simulink model "top_level_European_4segs_SR"  (R2025b)
settings: Solver=FixedStepAuto  StartTime=0.0  StopTime=tstop-Ts  RelTol=1e-3
undefined symbols (not defined in the file): DiscIntNeverNeededParam, dt, freq, idxC1, idxC2, idxC3, idxC4, n1, n2, n3, n4, Ts
libraries: eeRmsMeasurement x3
settings Model: SimulationMode=accelerator  Creator=gdudgeon  LastModifiedBy=gdudgeon
settings ModelReferenceCC: UpdateModelReferenceTargets=AssumeUpToDate  ParallelModelReferenceMATLABWorkerInit=Copy Base Workspace

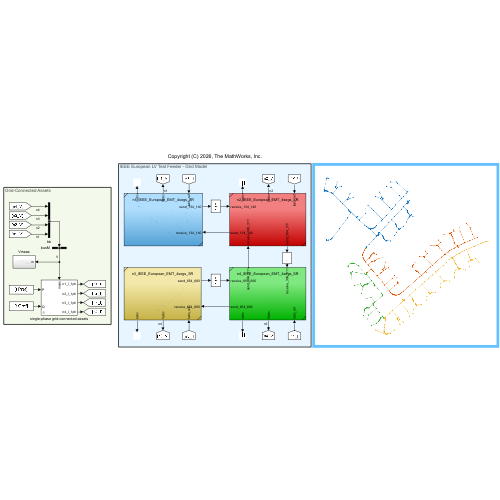
[thumbnail: Simulink's stored preview of the top-level diagram]
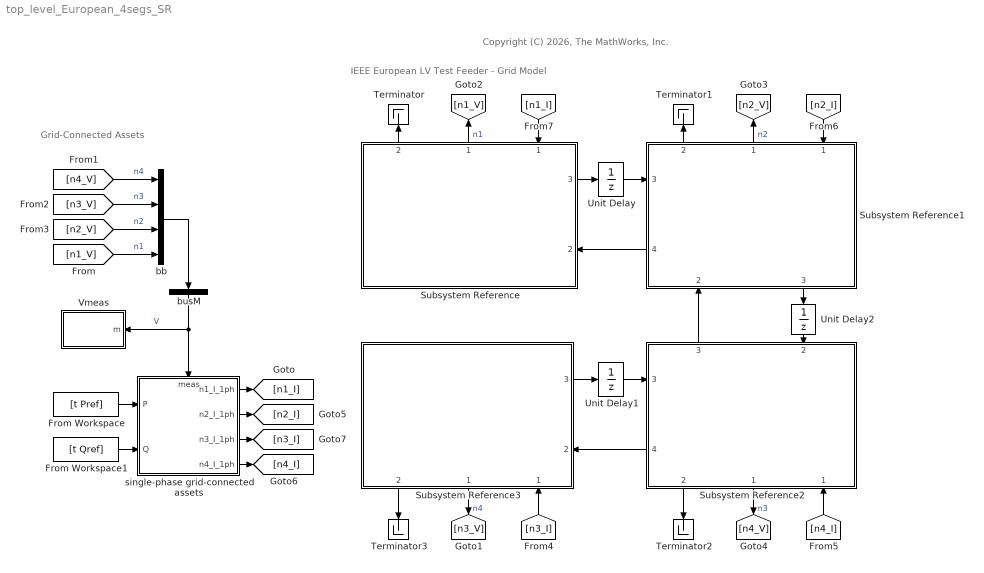
== system top_level_European_4segs_SR ==
  note: IEEE European LV Test Feeder - Grid Model
  note: Grid-Connected Assets
  note: Copyright (C) 2026, The MathWorks, Inc.
  From Workspace : FromWorkspace  VariableName=[t Pref]  SampleTime=Ts
  From Workspace1 : FromWorkspace  VariableName=[t Qref]  SampleTime=Ts
  Subsystem Reference : Subsystem  ReferencedSubsystem=n1_IEEE_European_EMT_4segs_SR
      settings: PortSchema="{\"entries\":[{\"content\":{\"sides\":[{\"content\":{},\"type\":\"ConnectorPlacement.EquallySpacedRectSide\",\"uuid\":\"0602a24e-b238-4b3f-aac8-5c5202892abf\"},{\"content\":{\"connectorIds\":[\"Out3\",\"In2\"],\"side\":\"RIGHT\"},\"type\":\"ConnectorPlacement.EquallySpacedRectSide\",\"uuid\":\"14efc789-be57-4299-a3a5-1e5073bae767\"},{\"content\":{\"connectorIds\":[\"Out2\",\"Out1\",\"In1\"],\"side\":\"TOP\"},\"type\":\"ConnectorPlacement.EquallySpacedRectSide\",\"uuid\":\"e86e604a-928b-4ba8-8b74-bfd217f971df\"}]},\"type\":\"ConnectorPlacement.EquallySpacedConnector\",\"uuid\":\"d0a53763-93a2-411e-b2ed-90390cf62489\"}],\"packageUris\":[\"http://schema.mathworks.com/mf0/Connector/R2020b\"],\"version\":\"1.0\"}"
  Subsystem Reference1 : Subsystem  ReferencedSubsystem=n2_IEEE_European_EMT_4segs_SR
      settings: PortSchema="{\"entries\":[{\"content\":{\"sides\":[{\"content\":{\"connectorIds\":[\"In3\",\"Out4\"]},\"type\":\"ConnectorPlacement.EquallySpacedRectSide\",\"uuid\":\"0602a24e-b238-4b3f-aac8-5c5202892abf\"},{\"content\":{\"side\":\"RIGHT\"},\"type\":\"ConnectorPlacement.EquallySpacedRectSide\",\"uuid\":\"14efc789-be57-4299-a3a5-1e5073bae767\"},{\"content\":{\"connectorIds\":[\"Out2\",\"Out1\",\"In1\"],\"side\":\"TOP\"},\"type\":\"ConnectorPlacement.EquallySpacedRectSide\",\"uuid\":\"e86e604a-928b-4ba8-8b74-bfd217f971df\"},{\"content\":{\"connectorIds\":[\"In2\",\"Out3\"],\"side\":\"BOTTOM\"},\"type\":\"ConnectorPlacement.EquallySpacedRectSide\",\"uuid\":\"6ffa862f-5c0a-45c7-b71b-4c92ac8f7e86\"}]},\"type\":\"ConnectorPlacement.EquallySpacedConnector\",\"uuid\":\"d0a53763-93a2-411e-b2ed-90390cf62489\"}],\"packageUris\":[\"http://schema.mathworks.com/mf0/Connector/R2020b\"],\"version\":\"1.0\"}"
  Subsystem Reference2 : Subsystem  ReferencedSubsystem=n4_IEEE_European_EMT_4segs_SR
      settings: PortSchema="{\"entries\":[{\"content\":{\"sides\":[{\"content\":{\"connectorIds\":[\"In3\",\"Out4\"]},\"type\":\"ConnectorPlacement.EquallySpacedRectSide\",\"uuid\":\"0602a24e-b238-4b3f-aac8-5c5202892abf\"},{\"content\":{\"side\":\"RIGHT\"},\"type\":\"ConnectorPlacement.EquallySpacedRectSide\",\"uuid\":\"14efc789-be57-4299-a3a5-1e5073bae767\"},{\"content\":{\"connectorIds\":[\"Out3\",\"In2\"],\"side\":\"TOP\"},\"type\":\"ConnectorPlacement.EquallySpacedRectSide\",\"uuid\":\"e86e604a-928b-4ba8-8b74-bfd217f971df\"},{\"content\":{\"connectorIds\":[\"Out2\",\"Out1\",\"In1\"],\"side\":\"BOTTOM\"},\"type\":\"ConnectorPlacement.EquallySpacedRectSide\",\"uuid\":\"6ffa862f-5c0a-45c7-b71b-4c92ac8f7e86\"}]},\"type\":\"ConnectorPlacement.EquallySpacedConnector\",\"uuid\":\"d0a53763-93a2-411e-b2ed-90390cf62489\"}],\"packageUris\":[\"http://schema.mathworks.com/mf0/Connector/R2020b\"],\"version\":\"1.0\"}"
  Subsystem Reference3 : Subsystem  ReferencedSubsystem=n3_IEEE_European_EMT_4segs_SR
      settings: PortSchema="{\"entries\":[{\"content\":{\"sides\":[{\"content\":{},\"type\":\"ConnectorPlacement.EquallySpacedRectSide\",\"uuid\":\"0602a24e-b238-4b3f-aac8-5c5202892abf\"},{\"content\":{\"connectorIds\":[\"Out3\",\"In2\"],\"side\":\"RIGHT\"},\"type\":\"ConnectorPlacement.EquallySpacedRectSide\",\"uuid\":\"14efc789-be57-4299-a3a5-1e5073bae767\"},{\"content\":{\"side\":\"TOP\"},\"type\":\"ConnectorPlacement.EquallySpacedRectSide\",\"uuid\":\"e86e604a-928b-4ba8-8b74-bfd217f971df\"},{\"content\":{\"connectorIds\":[\"Out2\",\"Out1\",\"In1\"],\"side\":\"BOTTOM\"},\"type\":\"ConnectorPlacement.EquallySpacedRectSide\",\"uuid\":\"6ffa862f-5c0a-45c7-b71b-4c92ac8f7e86\"}]},\"type\":\"ConnectorPlacement.EquallySpacedConnector\",\"uuid\":\"d0a53763-93a2-411e-b2ed-90390cf62489\"}],\"packageUris\":[\"http://schema.mathworks.com/mf0/Connector/R2020b\"],\"version\":\"1.0\"}"
  Terminator{,1..3} (4 alike) : Terminator
  Unit Delay : UnitDelay  SampleTime=-1  HasFrameUpgradeWarning=on
  Unit Delay1 : UnitDelay  SampleTime=-1  HasFrameUpgradeWarning=on
  Unit Delay2 : UnitDelay  SampleTime=-1  HasFrameUpgradeWarning=on
  Vmeas : Subsystem
  bb : BusCreator  Inputs=4
  busM : BusSelector  OutputSignals=n3.Vabc_660,n3.Vabc_666,n3.Vabc_672,n3.Vabc_673,n3.Vabc_679,n3.Vabc_680,n3.Vabc_685,n3.Vabc_686,n3.Vabc_689,n3.Vabc_690,n3.Vabc_691,n3.Vabc_693,n3.Vabc_694,n3.Vabc_695,n3.Vabc_696,n3.Vabc_697,n3.Vabc_699,n3.Vabc_700,n3.Vabc_701,n3.Vabc_702,n3.Vabc_703,n3.Vabc_705,n3.Vabc_706,n3.Vabc_707,n3.Vabc_708,n3.Vabc_710,n3.Vabc_711,n3.Vabc_712,n3.Vabc_713,n3.Vabc_714,n3.Vabc_716,n3.Vabc_717,n3.Vabc_718,n3.Vabc_719,n3.Vabc_720,n3.Vabc_722,n3.Vabc_723,n3.Vabc_724,n3.Vabc_725,n3.Vabc_726,n3.Vabc_727,n3.Vabc_729,n3.Vabc_730,n3.Vabc_731,n3.Vabc_732,n3.Vabc_733,n3.Vabc_734,n3.Vabc_736,n3.Vabc_737,n3.Vabc_738,n3.Vabc_739,n3.Vabc_740,n3.Vabc_741,n3.Vabc_743,n3.Vabc_744,n3.Vabc_745,n3.Vabc_746,n3.Vabc_747,n3.Vabc_748,n3.Vabc_749,n3.Vabc_751,n3.Vabc_752,n3.Vabc_753,n3.Vabc_754,n3.Vabc_755,n3.Vabc_756,n3.Vabc_757,n3.Vabc_758,n3.Vabc_760,n3.Vabc_761,n3.Vabc_762,n3.Vabc_763,n3.Vabc_764,n3.Vabc_765,n3.Vabc_766,n3.Vabc_768,n3.Vabc_769,n3.Vabc_770,n3.Vabc_771,n3.Vabc_772,n3.Vabc_773,n3.Vabc_774,n3.Vabc_775,n3.Vabc_777,n3.Vabc_778,n3.Vabc_779,n3.Vabc_780,n3.Vabc_781,n3.Vabc_782,n3.Vabc_783,n3.Vabc_784,n3.Vabc_786,n3.Vabc_787,n3.Vabc_788,n3.Vabc_789,n3.Vabc_790,n3.Vabc_791,n3.Vabc_792,n3.Vabc_793,n3.Vabc_794,n3.Vabc_795,n3.Vabc_796,n3.Vabc_797,n3.Vabc_798,n3.Vabc_799,n3.Vabc_800,n3.Vabc_801,n3.Vabc_802,n3.Vabc_803,n3.Vabc_804,n3.Vabc_805,n3.Vabc_806,n3.Vabc_807,n3.Vabc_808,n3.Vabc_809,n3.Vabc_810,n3.Vabc_811,n3.Vabc_812,n3.Vabc_813,n3.Vabc_814,n3.Vabc_815,n3.Vabc_816,n3.Vabc_817,n3.Vabc_818,n3.Vabc_819,n3.Vabc_820,n3.Vabc_821,n3.Vabc_822,n3.Vabc_823,n3.Vabc_824,n3.Vabc_825,n3.Vabc_826,n3.Vabc_827,n3.Vabc_828,n3.Vabc_829,n3.Vabc_830,n3.Vabc_831,n3.Vabc_832,n3.Vabc_833,n3.Vabc_834,n3.Vabc_835,n3.Vabc_836,n3.Vabc_837,n3.Vabc_838,n3.Vabc_839,n3.Vabc_840,n3.Vabc_841,n3.Vabc_842,n3.Vabc_843,n3.Vabc_844,n3.Vabc_845,n3.Vabc_846,n3.Vabc_847,n3.Vabc_848,n3.Vabc_849,n3.Vabc_850,n3.Vabc_851,n3.Vabc_852,n3.Vabc_853,n3.Vabc_854,n3.Vabc_855,n3.Vabc_856,n3.Vabc_857,n3.Vabc_858,n3.Vabc_859,n3.Vabc_860,n3.Vabc_861,n3.Vabc_862,n3.Vabc_863,n3.Vabc_864,n3.Vabc_865,n3.Vabc_866,n3.Vabc_867,n3.Vabc_868,n3.Vabc_869,n3.Vabc_870,n3.Vabc_871,n3.Vabc_872,n3.Vabc_873,n3.Vabc_874,n3.Vabc_875,n3.Vabc_876,n3.Vabc_877,n3.Vabc_878,n3.Vabc_879,n3.Vabc_880,n3.Vabc_881,n3.Vabc_882,n3.Vabc_883,n3.Vabc_884,n3.Vabc_885,n3.Vabc_886,n3.Vabc_887,n3.Vabc_888,n3.Vabc_889,n3.Vabc_890,n3.Vabc_891,n3.Vabc_892,n3.Vabc_893,n3.Vabc_894,n3.Vabc_895,n3.Vabc_896,n3.Vabc_897,n3.Vabc_898,n3.Vabc_899,n3.Vabc_900,n3.Vabc_901,n3.Vabc_902,n3.Vabc_903,n3.Vabc_904,n3.Vabc_905,n3.Vabc_906,n4.Vabc_311,n4.Vabc_319,n4.Vabc_326,n4.Vabc_333,n4.Vabc_340,n4.Vabc_347,n4.Vabc_353,n4.Vabc_358,n4.Vabc_363,n4.Vabc_368,n4.Vabc_373,n4.Vabc_378,n4.Vabc_379,n4.Vabc_384,n4.Vabc_385,n4.Vabc_386,n4.Vabc_391,n4.Vabc_392,n4.Vabc_393,n4.Vabc_396,n4.Vabc_397,n4.Vabc_398,n4.Vabc_399,n4.Vabc_402,n4.Vabc_403,n4.Vabc_404,n4.Vabc_405,n4.Vabc_408,n4.Vabc_409,n4.Vabc_410,n4.Vabc_411,n4.Vabc_412,n4.Vabc_414,n4.Vabc_415,n4.Vabc_416,n4.Vabc_417,n4.Vabc_418,n4.Vabc_420,n4.Vabc_421,n4.Vabc_422,n4.Vabc_423,n4.Vabc_424,n4.Vabc_427,n4.Vabc_428,n4.Vabc_429,n4.Vabc_430,n4.Vabc_431,n4.Vabc_434,n4.Vabc_435,n4.Vabc_436,n4.Vabc_437,n4.Vabc_438,n4.Vabc_441,n4.Vabc_442,n4.Vabc_443,n4.Vabc_444,n4.Vabc_445,n4.Vabc_448,n4.Vabc_449,n4.Vabc_450,n4.Vabc_451,n4.Vabc_452,n4.Vabc_455,n4.Vabc_456,n4.Vabc_457,n4.Vabc_458,n4.Vabc_459,n4.Vabc_463,n4.Vabc_464,n4.Vabc_465,n4.Vabc_466,n4.Vabc_471,n4.Vabc_472,n4.Vabc_473,n4.Vabc_474,n4.Vabc_478,n4.Vabc_479,n4.Vabc_480,n4.Vabc_481,n4.Vabc_486,n4.Vabc_487,n4.Vabc_488,n4.Vabc_489,n4.Vabc_495,n4.Vabc_496,n4.Vabc_497,n4.Vabc_498,n4.Vabc_504,n4.Vabc_505,n4.Vabc_506,n4.Vabc_507,n4.Vabc_512,n4.Vabc_513,n4.Vabc_514,n4.Vabc_515,n4.Vabc_521,n4.Vabc_522,n4.Vabc_523,n4.Vabc_524,n4.Vabc_530,n4.Vabc_531,n4.Vabc_532,n4.Vabc_538,n4.Vabc_539,n4.Vabc_540,n4.Vabc_541,n4.Vabc_547,n4.Vabc_548,n4.Vabc_549,n4.Vabc_556,n4.Vabc_557,n4.Vabc_558,n4.Vabc_565,n4.Vabc_566,n4.Vabc_572,n4.Vabc_578,n4.Vabc_585,n4.Vabc_586,n4.Vabc_593,n4.Vabc_594,n4.Vabc_601,n4.Vabc_602,n4.Vabc_603,n4.Vabc_613,n4.Vabc_614,n4.Vabc_615,n4.Vabc_623,n4.Vabc_624,n4.Vabc_625,n4.Vabc_630,n4.Vabc_631,n4.Vabc_632,n4.Vabc_636,n4.Vabc_637,n4.Vabc_638,n4.Vabc_642,n4.Vabc_643,n4.Vabc_644,n4.Vabc_647,n4.Vabc_648,n4.Vabc_649,n4.Vabc_652,n4.Vabc_653,n4.Vabc_654,n4.Vabc_658,n4.Vabc_659,n4.Vabc_664,n4.Vabc_665,n4.Vabc_670,n4.Vabc_671,n4.Vabc_677,n4.Vabc_678,n4.Vabc_683,n4.Vabc_684,n4.Vabc_687,n4.Vabc_688,n4.Vabc_692,n4.Vabc_698,n4.Vabc_704,n4.Vabc_709,n4.Vabc_715,n4.Vabc_721,n4.Vabc_728,n4.Vabc_735,n4.Vabc_742,n4.Vabc_750,n4.Vabc_759,n4.Vabc_767,n4.Vabc_776,n4.Vabc_785,n2.Vabc_140,n2.Vabc_146,n2.Vabc_153,n2.Vabc_160,n2.Vabc_168,n2.Vabc_177,n2.Vabc_186,n2.Vabc_195,n2.Vabc_205,n2.Vabc_215,n2.Vabc_224,n2.Vabc_232,n2.Vabc_240,n2.Vabc_247,n2.Vabc_255,n2.Vabc_256,n2.Vabc_262,n2.Vabc_263,n2.Vabc_270,n2.Vabc_271,n2.Vabc_272,n2.Vabc_278,n2.Vabc_279,n2.Vabc_280,n2.Vabc_285,n2.Vabc_286,n2.Vabc_287,n2.Vabc_288,n2.Vabc_294,n2.Vabc_295,n2.Vabc_296,n2.Vabc_297,n2.Vabc_301,n2.Vabc_302,n2.Vabc_303,n2.Vabc_304,n2.Vabc_308,n2.Vabc_309,n2.Vabc_310,n2.Vabc_315,n2.Vabc_316,n2.Vabc_317,n2.Vabc_318,n2.Vabc_322,n2.Vabc_323,n2.Vabc_324,n2.Vabc_325,n2.Vabc_328,n2.Vabc_329,n2.Vabc_330,n2.Vabc_331,n2.Vabc_332,n2.Vabc_334,n2.Vabc_335,n2.Vabc_336,n2.Vabc_337,n2.Vabc_338,n2.Vabc_339,n2.Vabc_341,n2.Vabc_342,n2.Vabc_343,n2.Vabc_344,n2.Vabc_345,n2.Vabc_346,n2.Vabc_348,n2.Vabc_349,n2.Vabc_350,n2.Vabc_351,n2.Vabc_352,n2.Vabc_354,n2.Vabc_355,n2.Vabc_356,n2.Vabc_357,n2.Vabc_359,n2.Vabc_360,n2.Vabc_361,n2.Vabc_362,n2.Vabc_364,n2.Vabc_365,n2.Vabc_366,n2.Vabc_367,n2.Vabc_369,n2.Vabc_370,n2.Vabc_371,n2.Vabc_372,n2.Vabc_374,n2.Vabc_375,n2.Vabc_376,n2.Vabc_377,n2.Vabc_380,n2.Vabc_381,n2.Vabc_382,n2.Vabc_383,n2.Vabc_387,n2.Vabc_388,n2.Vabc_389,n2.Vabc_390,n2.Vabc_394,n2.Vabc_395,n2.Vabc_400,n2.Vabc_401,n2.Vabc_406,n2.Vabc_407,n2.Vabc_413,n2.Vabc_419,n2.Vabc_425,n2.Vabc_426,n2.Vabc_432,n2.Vabc_433,n2.Vabc_439,n2.Vabc_440,n2.Vabc_446,n2.Vabc_447,n2.Vabc_453,n2.Vabc_454,n2.Vabc_460,n2.Vabc_461,n2.Vabc_462,n2.Vabc_467,n2.Vabc_468,n2.Vabc_469,n2.Vabc_470,n2.Vabc_475,n2.Vabc_476,n2.Vabc_477,n2.Vabc_482,n2.Vabc_483,n2.Vabc_484,n2.Vabc_485,n2.Vabc_490,n2.Vabc_491,n2.Vabc_492,n2.Vabc_493,n2.Vabc_494,n2.Vabc_499,n2.Vabc_500,n2.Vabc_501,n2.Vabc_502,n2.Vabc_503,n2.Vabc_508,n2.Vabc_509,n2.Vabc_510,n2.Vabc_511,n2.Vabc_516,n2.Vabc_517,n2.Vabc_518,n2.Vabc_519,n2.Vabc_520,n2.Vabc_525,n2.Vabc_526,n2.Vabc_527,n2.Vabc_528,n2.Vabc_529,n2.Vabc_533,n2.Vabc_534,n2.Vabc_535,n2.Vabc_536,n2.Vabc_537,n2.Vabc_542,n2.Vabc_543,n2.Vabc_544,n2.Vabc_545,n2.Vabc_546,n2.Vabc_550,n2.Vabc_551,n2.Vabc_552,n2.Vabc_553,n2.Vabc_554,n2.Vabc_555,n2.Vabc_559,n2.Vabc_560,n2.Vabc_561,n2.Vabc_562,n2.Vabc_563,n2.Vabc_564,n2.Vabc_567,n2.Vabc_568,n2.Vabc_569,n2.Vabc_570,n2.Vabc_571,n2.Vabc_573,n2.Vabc_574,n2.Vabc_575,n2.Vabc_576,n2.Vabc_577,n2.Vabc_579,n2.Vabc_580,n2.Vabc_581,n2.Vabc_582,n2.Vabc_583,n2.Vabc_584,n2.Vabc_587,n2.Vabc_588,n2.Vabc_589,n2.Vabc_590,n2.Vabc_591,n2.Vabc_592,n2.Vabc_595,n2.Vabc_596,n2.Vabc_597,n2.Vabc_598,n2.Vabc_599,n2.Vabc_600,n2.Vabc_604,n2.Vabc_605,n2.Vabc_606,n2.Vabc_607,n2.Vabc_608,n2.Vabc_609,n2.Vabc_610,n2.Vabc_611,n2.Vabc_612,n2.Vabc_616,n2.Vabc_617,n2.Vabc_618,n2.Vabc_619,n2.Vabc_620,n2.Vabc_621,n2.Vabc_622,n2.Vabc_626,n2.Vabc_627,n2.Vabc_628,n2.Vabc_629,n2.Vabc_633,n2.Vabc_634,n2.Vabc_635,n2.Vabc_639,n2.Vabc_640,n2.Vabc_641,n2.Vabc_645,n2.Vabc_646,n2.Vabc_650,n2.Vabc_651,n2.Vabc_655,n2.Vabc_656,n2.Vabc_657,n2.Vabc_661,n2.Vabc_662,n2.Vabc_663,n2.Vabc_667,n2.Vabc_668,n2.Vabc_669,n2.Vabc_674,n2.Vabc_675,n2.Vabc_676,n2.Vabc_681,n2.Vabc_682,n1.Vabc_1,n1.Vabc_10,n1.Vabc_100,n1.Vabc_101,n1.Vabc_102,n1.Vabc_103,n1.Vabc_104,n1.Vabc_105,n1.Vabc_106,n1.Vabc_107,n1.Vabc_108,n1.Vabc_109,n1.Vabc_11,n1.Vabc_110,n1.Vabc_111,n1.Vabc_112,n1.Vabc_113,n1.Vabc_114,n1.Vabc_115,n1.Vabc_116,n1.Vabc_117,n1.Vabc_118,n1.Vabc_119,n1.Vabc_12,n1.Vabc_120,n1.Vabc_121,n1.Vabc_122,n1.Vabc_123,n1.Vabc_124,n1.Vabc_125,n1.Vabc_126,n1.Vabc_127,n1.Vabc_128,n1.Vabc_129,n1.Vabc_13,n1.Vabc_130,n1.Vabc_131,n1.Vabc_132,n1.Vabc_133,n1.Vabc_134,n1.Vabc_135,n1.Vabc_136,n1.Vabc_137,n1.Vabc_138,n1.Vabc_139,n1.Vabc_14,n1.Vabc_141,n1.Vabc_142,n1.Vabc_143,n1.Vabc_144,n1.Vabc_145,n1.Vabc_147,n1.Vabc_148,n1.Vabc_149,n1.Vabc_15,n1.Vabc_150,n1.Vabc_151,n1.Vabc_152,n1.Vabc_154,n1.Vabc_155,n1.Vabc_156,n1.Vabc_157,n1.Vabc_158,n1.Vabc_159,n1.Vabc_16,n1.Vabc_161,n1.Vabc_162,n1.Vabc_163,n1.Vabc_164,n1.Vabc_165,n1.Vabc_166,n1.Vabc_167,n1.Vabc_169,n1.Vabc_17,n1.Vabc_170,n1.Vabc_171,n1.Vabc_172,n1.Vabc_173,n1.Vabc_174,n1.Vabc_175,n1.Vabc_176,n1.Vabc_178,n1.Vabc_179,n1.Vabc_18,n1.Vabc_180,n1.Vabc_181,n1.Vabc_182,n1.Vabc_183,n1.Vabc_184,n1.Vabc_185,n1.Vabc_187,n1.Vabc_188,n1.Vabc_189,n1.Vabc_19,n1.Vabc_190,n1.Vabc_191,n1.Vabc_192,n1.Vabc_193,n1.Vabc_194,n1.Vabc_196,n1.Vabc_197,n1.Vabc_198,n1.Vabc_199,n1.Vabc_2,n1.Vabc_20,n1.Vabc_200,n1.Vabc_201,n1.Vabc_202,n1.Vabc_203,n1.Vabc_204,n1.Vabc_206,n1.Vabc_207,n1.Vabc_208,n1.Vabc_209,n1.Vabc_21,n1.Vabc_210,n1.Vabc_211,n1.Vabc_212,n1.Vabc_213,n1.Vabc_214,n1.Vabc_216,n1.Vabc_217,n1.Vabc_218,n1.Vabc_219,n1.Vabc_22,n1.Vabc_220,n1.Vabc_221,n1.Vabc_222,n1.Vabc_223,n1.Vabc_225,n1.Vabc_226,n1.Vabc_227,n1.Vabc_228,n1.Vabc_229,n1.Vabc_23,n1.Vabc_230,n1.Vabc_231,n1.Vabc_233,n1.Vabc_234,n1.Vabc_235,n1.Vabc_236,n1.Vabc_237,n1.Vabc_238,n1.Vabc_239,n1.Vabc_24,n1.Vabc_241,n1.Vabc_242,n1.Vabc_243,n1.Vabc_244,n1.Vabc_245,n1.Vabc_246,n1.Vabc_248,n1.Vabc_249,n1.Vabc_25,n1.Vabc_250,n1.Vabc_251,n1.Vabc_252,n1.Vabc_253,n1.Vabc_254,n1.Vabc_257,n1.Vabc_258,n1.Vabc_259,n1.Vabc_26,n1.Vabc_260,n1.Vabc_261,n1.Vabc_264,n1.Vabc_265,n1.Vabc_266,n1.Vabc_267,n1.Vabc_268,n1.Vabc_269,n1.Vabc_27,n1.Vabc_273,n1.Vabc_274,n1.Vabc_275,n1.Vabc_276,n1.Vabc_277,n1.Vabc_28,n1.Vabc_281,n1.Vabc_282,n1.Vabc_283,n1.Vabc_284,n1.Vabc_289,n1.Vabc_29,n1.Vabc_290,n1.Vabc_291,n1.Vabc_292,n1.Vabc_293,n1.Vabc_298,n1.Vabc_299,n1.Vabc_3,n1.Vabc_30,n1.Vabc_300,n1.Vabc_305,n1.Vabc_306,n1.Vabc_307,n1.Vabc_31,n1.Vabc_312,n1.Vabc_313,n1.Vabc_314,n1.Vabc_32,n1.Vabc_320,n1.Vabc_321,n1.Vabc_327,n1.Vabc_33,n1.Vabc_34,n1.Vabc_35,n1.Vabc_36,n1.Vabc_37,n1.Vabc_38,n1.Vabc_39,n1.Vabc_4,n1.Vabc_40,n1.Vabc_41,n1.Vabc_42,n1.Vabc_43,n1.Vabc_44,n1.Vabc_45,n1.Vabc_46,n1.Vabc_47,n1.Vabc_48,n1.Vabc_49,n1.Vabc_5,n1.Vabc_50,n1.Vabc_51,n1.Vabc_52,n1.Vabc_53,n1.Vabc_54,n1.Vabc_55,n1.Vabc_56,n1.Vabc_57,n1.Vabc_58,n1.Vabc_59,n1.Vabc_6,n1.Vabc_60,n1.Vabc_61,n1.Vabc_62,n1.Vabc_63,n1.Vabc_64,n1.Vabc_65,n1.Vabc_66,n1.Vabc_67,n1.Vabc_68,n1.Vabc_69,n1.Vabc_7,n1.Vabc_70,n1.Vabc_71,n1.Vabc_72,n1.Vabc_73,n1.Vabc_74,n1.Vabc_75,n1.Vabc_76,n1.Vabc_77,n1.Vabc_78,n1.Vabc_79,n1.Vabc_8,n1.Vabc_80,n1.Vabc_81,n1.Vabc_82,n1.Vabc_83,n1.Vabc_84,n1.Vabc_85,n1.Vabc_86,n1.Vabc_87,n1.Vabc_88,n1.Vabc_89,n1.Vabc_9,n1.Vabc_90,n1.Vabc_91,n1.Vabc_92,n1.Vabc_93,n1.Vabc_94,n1.Vabc_95,n1.Vabc_96,n1.Vabc_97,n1.Vabc_98,n1.Vabc_99  OutputAsBus=on
  single-phase grid-connected assets : Subsystem  mask{num_loads=55}
      mask prompts: num_loads "Number of loads"
      settings: PortSchema="{\"entries\":[{\"content\":{\"sides\":[{\"content\":{\"connectorIds\":[\"In1\",\"In2\"]},\"type\":\"ConnectorPlacement.EquallySpacedRectSide\",\"uuid\":\"dcb77ad6-d65a-4afe-9b75-44cea2e03bc8\"},{\"content\":{\"connectorIds\":[\"Out1\",\"Out2\",\"Out3\",\"Out4\"],\"side\":\"RIGHT\"},\"type\":\"ConnectorPlacement.EquallySpacedRectSide\",\"uuid\":\"20550ec8-912f-4e6b-8efc-55d7f6680ac4\"},{\"content\":{\"connectorIds\":[\"In3\"],\"side\":\"TOP\"},\"type\":\"ConnectorPlacement.EquallySpacedRectSide\",\"uuid\":\"6ad8cbf4-1495-4620-97d9-4b8af34d00d1\"}]},\"type\":\"ConnectorPlacement.EquallySpacedConnector\",\"uuid\":\"b57ec49b-aa32-43b3-a026-14ed90072d63\"}],\"packageUris\":[\"http://schema.mathworks.com/mf0/Connector/R2020b\"],\"version\":\"1.0\"}"
  wires:
  From Workspace1/1 -> single-phase grid-connected assets/2(Q)
  From Workspace/1 -> single-phase grid-connected assets/1(P)
  Subsystem Reference/2 -> Terminator/1
  Subsystem Reference1/2 -> Terminator1/1
  bb/1 -> busM/1
  busM/1 -> Vmeas/1(m), single-phase grid-connected assets/3(meas)  "V"
  Subsystem Reference/3 -> Unit Delay/1
  Subsystem Reference1/3 -> Unit Delay2/1
  Unit Delay/1 -> Subsystem Reference1/3
  Subsystem Reference1/4 -> Subsystem Reference/2
  Unit Delay2/1 -> Subsystem Reference2/2
  Subsystem Reference2/3 -> Subsystem Reference1/2
  Subsystem Reference2/2 -> Terminator2/1
  Subsystem Reference3/2 -> Terminator3/1
  Subsystem Reference3/3 -> Unit Delay1/1
  Subsystem Reference2/4 -> Subsystem Reference3/2
  [n1_V] -> bb/4  "n1"
  [n4_V] -> bb/1  "n4"
  [n3_V] -> bb/2  "n3"
  [n2_V] -> bb/3  "n2"
  Subsystem Reference2/1 -> [n4_V]  "n3"
  Subsystem Reference3/1 -> [n3_V]  "n4"
  Subsystem Reference1/1 -> [n2_V]  "n2"
  Subsystem Reference/1 -> [n1_V]  "n1"
  Unit Delay1/1 -> Subsystem Reference2/3
  single-phase grid-connected assets/1(n1_I_1ph) -> [n1_I]
  single-phase grid-connected assets/2(n2_I_1ph) -> [n2_I]
  single-phase grid-connected assets/3(n3_I_1ph) -> [n3_I]
  single-phase grid-connected assets/4(n4_I_1ph) -> [n4_I]
  [n3_I] -> Subsystem Reference3/1
  [n2_I] -> Subsystem Reference1/1
  [n1_I] -> Subsystem Reference/1
  [n4_I] -> Subsystem Reference2/1

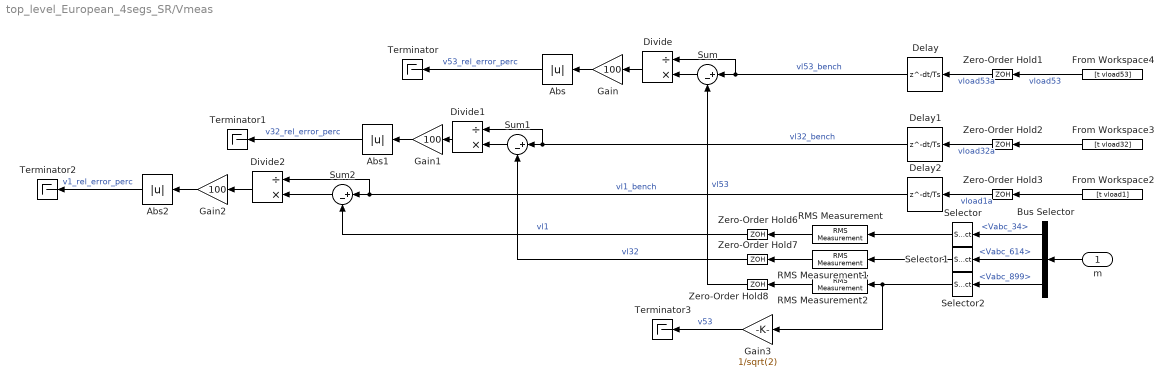
== system top_level_European_4segs_SR/Vmeas ==
  m : Inport
  Abs : Abs  SaturateOnIntegerOverflow=off
  Abs1 : Abs  SaturateOnIntegerOverflow=off
  Abs2 : Abs  SaturateOnIntegerOverflow=off
  Bus Selector : BusSelector  OutputSignals=Vabc_34,Vabc_614,Vabc_899
  Delay : Delay  DelayLength=dt/Ts  SampleTime=Ts
  Delay1 : Delay  DelayLength=dt/Ts  SampleTime=Ts
  Delay2 : Delay  DelayLength=dt/Ts  SampleTime=Ts
  Divide : Product  Inputs=/*
  Divide1 : Product  Inputs=/*
  Divide2 : Product  Inputs=/*
  From Workspace2 : FromWorkspace  VariableName=[t vload1]  SampleTime=Ts
  From Workspace3 : FromWorkspace  VariableName=[t vload32]  SampleTime=Ts
  From Workspace4 : FromWorkspace  VariableName=[t vload53]  SampleTime=Ts
  Gain : Gain  Gain=100
  Gain1 : Gain  Gain=100
  Gain2 : Gain  Gain=100
  Gain3 : Gain  Gain=1/sqrt(2)
  RMS Measurement : eeRmsMeasurement/RMS Measurement  LabelModeActiveChoice=Total  F=freq  SpecifyHarmonics=off  K=[0 1 2]  Ts=Ts
      settings: LibrarySourceBlock=|
      | ee_sl_lib/Measurements/RMS
      | Measurement
  RMS Measurement1 : eeRmsMeasurement/RMS Measurement  LabelModeActiveChoice=Total  F=freq  SpecifyHarmonics=off  K=[0 1 2]  Ts=Ts
      settings: LibrarySourceBlock=|
      | ee_sl_lib/Measurements/RMS
      | Measurement
  RMS Measurement2 : eeRmsMeasurement/RMS Measurement  LabelModeActiveChoice=Total  F=freq  SpecifyHarmonics=off  K=[0 1 2]  Ts=Ts
      settings: LibrarySourceBlock=|
      | ee_sl_lib/Measurements/RMS
      | Measurement
  Selector : Selector  InputPortWidth=3  IndexOptions=Index vector (dialog)  Indices=1  OutputSizes=1
  Selector1 : Selector  InputPortWidth=3  IndexOptions=Index vector (dialog)  Indices=3  OutputSizes=1
  Selector2 : Selector  InputPortWidth=3  IndexOptions=Index vector (dialog)  Indices=2  OutputSizes=1
  Sum : Sum  Inputs=|+-
  Sum1 : Sum  Inputs=|+-
  Sum2 : Sum  Inputs=|+-
  Terminator{,1..3} (4 alike) : Terminator
  Zero-Order Hold{1..3,6..8} (6 alike) : ZeroOrderHold  SampleTime=dt
  wires:
  Zero-Order Hold3/1 -> Delay2/1  "vload1a"
  Zero-Order Hold2/1 -> Delay1/1  "vload32a"
  Zero-Order Hold1/1 -> Delay/1  "vload53a"
  From Workspace2/1 -> Zero-Order Hold3/1
  From Workspace3/1 -> Zero-Order Hold2/1
  From Workspace4/1 -> Zero-Order Hold1/1  "vload53"
  Gain3/1 -> Terminator3/1  "v53"
  Zero-Order Hold8/1 -> Sum/2  "vl53"
  Zero-Order Hold7/1 -> Sum1/2  "vl32"
  Zero-Order Hold6/1 -> Sum2/2  "vl1"
  Abs2/1 -> Terminator2/1  "v1_rel_error_perc"
  Abs1/1 -> Terminator1/1  "v32_rel_error_perc"
  Abs/1 -> Terminator/1  "v53_rel_error_perc"
  Gain2/1 -> Abs2/1
  Gain1/1 -> Abs1/1
  Gain/1 -> Abs/1
  Divide1/1 -> Gain1/1
  RMS Measurement2/1 -> Zero-Order Hold8/1
  RMS Measurement1/1 -> Zero-Order Hold7/1
  RMS Measurement/1 -> Zero-Order Hold6/1
  Divide/1 -> Gain/1
  Divide2/1 -> Gain2/1
  Sum/1 -> Divide/2
  Sum1/1 -> Divide1/2
  Sum2/1 -> Divide2/2
  m/1 -> Bus Selector/1
  Bus Selector/3 -> Selector2/1  "<Vabc_899>"
  Selector/1 -> RMS Measurement/1
  Bus Selector/1 -> Selector/1  "<Vabc_34>"
  Selector1/1 -> RMS Measurement1/1
  Bus Selector/2 -> Selector1/1  "<Vabc_614>"
  Delay/1 -> Sum/1, Divide/1  "vl53_bench"
  Selector2/1 -> RMS Measurement2/1, Gain3/1
  Delay1/1 -> Sum1/1, Divide1/1  "vl32_bench"
  Delay2/1 -> Sum2/1, Divide2/1  "vl1_bench"

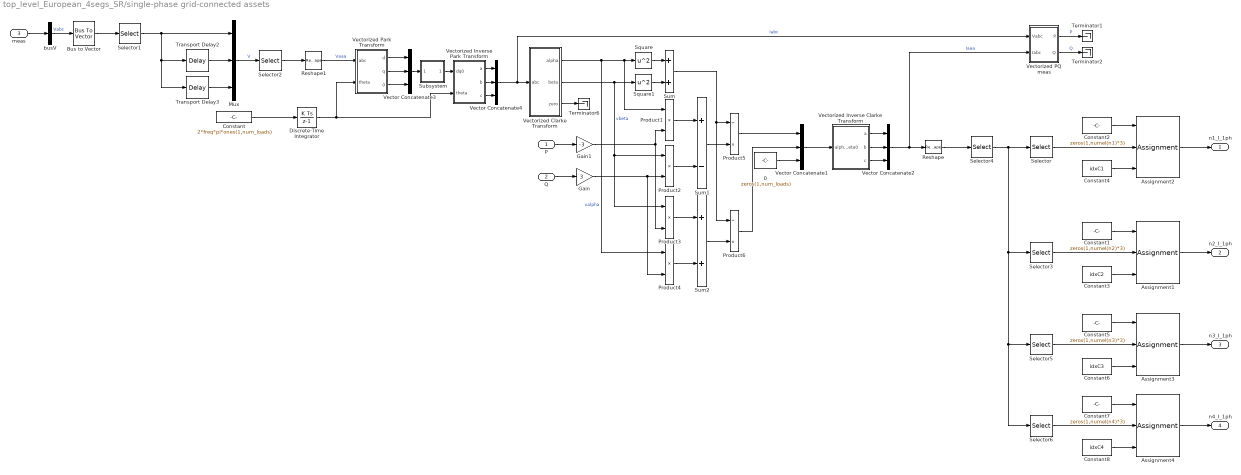
== system top_level_European_4segs_SR/single-phase grid-connected assets ==
  P : Inport
  Q : Inport  Port=2
  meas : Inport  Port=3
  "0 " : Constant  Value=zeros(1,num_loads)  VectorParams1D=off  SampleTime=Ts
  Assignment{1..4} (4 alike) : Assignment  IndexOptions=Index vector (port)  Indices=1  OutputSizes=1
  Bus to Vector : BusToVector
  Constant : Constant  Value=2*freq*pi*ones(1,num_loads)  VectorParams1D=off  SampleTime=Ts
  Constant1 : Constant  Value=zeros(1,numel(n2)*3)  SampleTime=Ts
  Constant2 : Constant  Value=zeros(1,numel(n1)*3)  SampleTime=Ts
  Constant3 : Constant  Value=idxC2  SampleTime=Ts
  Constant4 : Constant  Value=idxC1  SampleTime=Ts
  Constant5 : Constant  Value=zeros(1,numel(n3)*3)  SampleTime=Ts
  Constant6 : Constant  Value=idxC3  SampleTime=Ts
  Constant7 : Constant  Value=zeros(1,numel(n4)*3)  SampleTime=Ts
  Constant8 : Constant  Value=idxC4  SampleTime=Ts
  Discrete-Time Integrator : DiscreteIntegrator  SampleTime=Ts  ICPrevOutput=DiscIntNeverNeededParam  ICPrevScaledInput=DiscIntNeverNeededParam
  Gain : Gain  Gain=3
  Gain1 : Gain  Gain=-3
  Mux : Mux  Inputs=3
  Product{1..4} (4 alike) : Product
  Product5 : Product  Inputs=/*
  Product6 : Product  Inputs=/*
  Reshape : Reshape
  Reshape1 : Reshape  OutputDimensionality=Customize  OutputDimensions=[3,num_loads]
  Selector : Selector  InputPortWidth=55  IndexOptions=Index vector (dialog)  Indices=idx_n1  OutputSizes=1
  Selector1 : Selector  InputPortWidth=55*3  IndexOptions=Index vector (dialog)  Indices=idxLoads  OutputSizes=1
  Selector2 : Selector  InputPortWidth=165  IndexOptions=Index vector (dialog)  Indices=idxR  OutputSizes=1
  Selector3 : Selector  InputPortWidth=55  IndexOptions=Index vector (dialog)  Indices=idx_n2  OutputSizes=1
  Selector4 : Selector  InputPortWidth=165  IndexOptions=Index vector (dialog)  Indices=1:3:165  OutputSizes=1
  Selector5 : Selector  InputPortWidth=55  IndexOptions=Index vector (dialog)  Indices=idx_n3  OutputSizes=1
  Selector6 : Selector  InputPortWidth=55  IndexOptions=Index vector (dialog)  Indices=idx_n4  OutputSizes=1
  Square : Math  Operator=square
  Square1 : Math  Operator=square
  Subsystem : Subsystem
  Sum : Sum
  Sum1 : Sum  Inputs=+-
  Sum2 : Sum
  Terminator1 : Terminator
  Terminator2 : Terminator
  Terminator6 : Terminator
  Transport Delay2 : TransportDelay  DelayTime=1/3/freq
  Transport Delay3 : TransportDelay  DelayTime=2/3/freq
  Vector Concatenate{1..4} (4 alike) : Concatenate  NumInputs=3  Mode=Multidimensional array
  Vectorized Clarke Transform : Subsystem  mask{no_meas=num_loads}
      mask prompts: no_meas "Number of measurements"
  Vectorized PQ meas : Subsystem  DialogController=POWERSYS.PowerSysDialog
  Vectorized Park Transform : Subsystem  mask{no_meas=num_loads}
      mask prompts: no_meas "Number of measurements"
  Vectorized Inverse Clarke Transform : Subsystem  mask{no_meas=num_loads}
      mask prompts: no_meas "Number of Measurements"
      mask Display:
      | port_label('input', 1, '\alpha\beta0', 'texmode', 'on')
      | port_label('output',1,'a')
      | port_label('output',2,'b')
      | port_label('output',3,'c')
  Vectorized Inverse Park Transform : Subsystem  mask{no_meas=num_loads}
      mask prompts: no_meas "Number of Measurements"
  busV : BusSelector  OutputSignals=Vabc_34,Vabc_47,Vabc_70,Vabc_73,Vabc_74,Vabc_83,Vabc_178,Vabc_208,Vabc_225,Vabc_248,Vabc_249,Vabc_264,Vabc_276,Vabc_289,Vabc_314,Vabc_320,Vabc_327,Vabc_337,Vabc_342,Vabc_349,Vabc_387,Vabc_388,Vabc_406,Vabc_458,Vabc_502,Vabc_522,Vabc_539,Vabc_556,Vabc_562,Vabc_563,Vabc_611,Vabc_614,Vabc_619,Vabc_629,Vabc_639,Vabc_676,Vabc_682,Vabc_688,Vabc_701,Vabc_702,Vabc_755,Vabc_778,Vabc_780,Vabc_785,Vabc_813,Vabc_817,Vabc_835,Vabc_860,Vabc_861,Vabc_886,Vabc_896,Vabc_898,Vabc_899,Vabc_900,Vabc_906  OutputAsBus=on
  n1_I_1ph : Outport
  n2_I_1ph : Outport  Port=2
  n3_I_1ph : Outport  Port=3
  n4_I_1ph : Outport  Port=4
  wires:
  Selector2/1 -> Reshape1/1
  Mux/1 -> Selector2/1  "V"
  Reshape1/1 -> Vectorized Park Transform/1(abc)  "Vaaa"
  Transport Delay2/1 -> Mux/2
  Transport Delay3/1 -> Mux/3
  Assignment2/1 -> n1_I_1ph/1
  Selector1/1 -> Transport Delay3/1, Transport Delay2/1, Mux/1
  busV/1 -> Bus to Vector/1  "Vabc"
  Constant4/1 -> Assignment2/3
  Constant2/1 -> Assignment2/1
  Gain1/1 -> Product3/2, Product1/2
  Gain/1 -> Product2/2, Product4/2
  Bus to Vector/1 -> Selector1/1
  Subsystem/1(Out1) -> Vectorized Inverse Park Transform/1(dq0)
  Vector Concatenate3/1 -> Subsystem/1(In1)
  Discrete-Time Integrator/1 -> Vectorized Park Transform/2(theta), Vectorized Inverse Park Transform/2(theta)
  Constant/1 -> Discrete-Time Integrator/1
  Vector Concatenate4/1 -> Vectorized PQ meas/1(Vabc), Vectorized Clarke Transform/1(abc)  "Iabc"
  Vectorized Inverse Park Transform/3(c) -> Vector Concatenate4/3
  Vectorized Inverse Park Transform/2(b) -> Vector Concatenate4/2
  Vectorized Inverse Park Transform/1(a) -> Vector Concatenate4/1
  Vectorized Park Transform/3(0) -> Vector Concatenate3/3
  Vectorized Park Transform/2(q) -> Vector Concatenate3/2
  Vectorized Park Transform/1(d) -> Vector Concatenate3/1
  Vector Concatenate2/1 -> Vectorized PQ meas/2(Iabc), Reshape/1  "Iaaa"
  Vectorized PQ meas/2(Q) -> Terminator2/1  "Q"
  Vectorized PQ meas/1(P) -> Terminator1/1  "P"
  Product5/1 -> Vector Concatenate1/1
  Square/1 -> Sum/1
  Vector Concatenate1/1 -> Vectorized Inverse Clarke Transform/1(alphabeta0)
  meas/1 -> busV/1
  Product1/1 -> Sum1/1
  Vectorized Inverse Clarke Transform/3(c) -> Vector Concatenate2/3
  Product4/1 -> Sum2/2
  Product6/1 -> Vector Concatenate1/2
  Vectorized Clarke Transform/1(alpha) -> Square/1, Product1/1, Product4/1  "valpha"
  Product2/1 -> Sum1/2
  Vectorized Clarke Transform/3(zero) -> Terminator6/1
  Vectorized Inverse Clarke Transform/2(b) -> Vector Concatenate2/2
  Vectorized Inverse Clarke Transform/1(a) -> Vector Concatenate2/1
  Sum1/1 -> Product5/2
  "0 "/1 -> Vector Concatenate1/3
  Q/1 -> Gain/1
  Vectorized Clarke Transform/2(beta) -> Square1/1, Product2/1, Product3/1  "vbeta"
  Product3/1 -> Sum2/1
  Square1/1 -> Sum/2
  P/1 -> Gain1/1
  Sum/1 -> Product6/1, Product5/1
  Sum2/1 -> Product6/2
  Reshape/1 -> Selector4/1
  Constant1/1 -> Assignment1/1
  Constant3/1 -> Assignment1/3
  Assignment1/1 -> n2_I_1ph/1
  Selector4/1 -> Selector/1, Selector6/1, Selector5/1, Selector3/1
  Selector/1 -> Assignment2/2
  Selector3/1 -> Assignment1/2
  Selector5/1 -> Assignment3/2
  Assignment3/1 -> n3_I_1ph/1
  Constant6/1 -> Assignment3/3
  Constant5/1 -> Assignment3/1
  Constant7/1 -> Assignment4/1
  Constant8/1 -> Assignment4/3
  Assignment4/1 -> n4_I_1ph/1
  Selector6/1 -> Assignment4/2

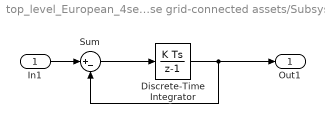
== system top_level_European_4segs_SR/single-phase grid-connected assets/Subsystem ==
  In1 : Inport
  Discrete-Time Integrator : DiscreteIntegrator  gainval=100  InitialCondition=1  SampleTime=-1  ICPrevOutput=DiscIntNeverNeededParam  ICPrevScaledInput=DiscIntNeverNeededParam
  Sum : Sum  Inputs=|+-
  Out1 : Outport
  wires:
  Discrete-Time Integrator/1 -> Out1/1, Sum/2
  Sum/1 -> Discrete-Time Integrator/1
  In1/1 -> Sum/1

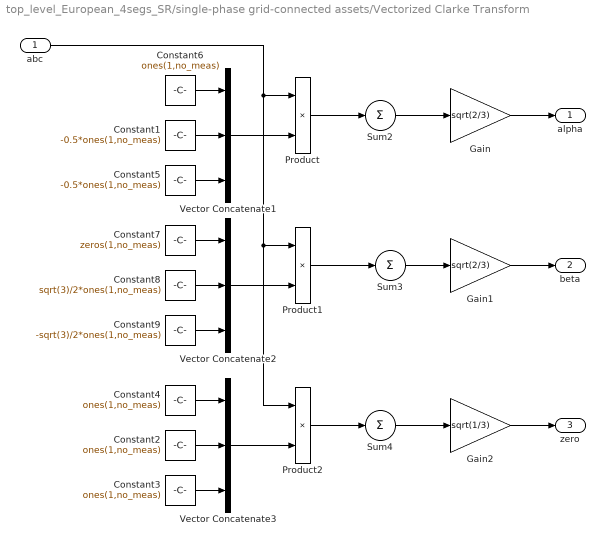
== system top_level_European_4segs_SR/single-phase grid-connected assets/Vectorized Clarke Transform ==
  abc : Inport
  Constant1 : Constant  Value=-0.5*ones(1,no_meas)  VectorParams1D=off  SampleTime=Ts
  Constant{2..4,6} (4 alike) : Constant  Value=ones(1,no_meas)  VectorParams1D=off  SampleTime=Ts
  Constant5 : Constant  Value=-0.5*ones(1,no_meas)  VectorParams1D=off  SampleTime=Ts
  Constant7 : Constant  Value=zeros(1,no_meas)  VectorParams1D=off  SampleTime=Ts
  Constant8 : Constant  Value=sqrt(3)/2*ones(1,no_meas)  VectorParams1D=off  SampleTime=Ts
  Constant9 : Constant  Value=-sqrt(3)/2*ones(1,no_meas)  VectorParams1D=off  SampleTime=Ts
  Gain : Gain  Gain=sqrt(2/3)
  Gain1 : Gain  Gain=sqrt(2/3)
  Gain2 : Gain  Gain=sqrt(1/3)
  Product : Product
  Product1 : Product
  Product2 : Product
  Sum2 : Sum  Inputs=1  CollapseMode=Specified dimension  InputSameDT=on  SaturateOnIntegerOverflow=on  OutDataTypeStr=Inherit: Same as first input
  Sum3 : Sum  Inputs=1  CollapseMode=Specified dimension  InputSameDT=on  SaturateOnIntegerOverflow=on  OutDataTypeStr=Inherit: Same as first input
  Sum4 : Sum  Inputs=1  CollapseMode=Specified dimension  InputSameDT=on  SaturateOnIntegerOverflow=on  OutDataTypeStr=Inherit: Same as first input
  Vector Concatenate1 : Concatenate  NumInputs=3  Mode=Multidimensional array
  Vector Concatenate2 : Concatenate  NumInputs=3  Mode=Multidimensional array
  Vector Concatenate3 : Concatenate  NumInputs=3  Mode=Multidimensional array
  alpha : Outport  VectorParamsAs1DForOutWhenUnconnected=off
  beta : Outport  Port=2  VectorParamsAs1DForOutWhenUnconnected=off
  zero : Outport  Port=3  VectorParamsAs1DForOutWhenUnconnected=off
  wires:
  Constant9/1 -> Vector Concatenate2/3
  Constant8/1 -> Vector Concatenate2/2
  Constant7/1 -> Vector Concatenate2/1
  Constant5/1 -> Vector Concatenate1/3
  Constant1/1 -> Vector Concatenate1/2
  Constant6/1 -> Vector Concatenate1/1
  abc/1 -> Product2/1, Product1/1, Product/1
  Constant4/1 -> Vector Concatenate3/1
  Constant2/1 -> Vector Concatenate3/2
  Constant3/1 -> Vector Concatenate3/3
  Vector Concatenate3/1 -> Product2/2
  Vector Concatenate2/1 -> Product1/2
  Vector Concatenate1/1 -> Product/2
  Product/1 -> Sum2/1
  Product1/1 -> Sum3/1
  Product2/1 -> Sum4/1
  Sum3/1 -> Gain1/1
  Sum4/1 -> Gain2/1
  Sum2/1 -> Gain/1
  Gain2/1 -> zero/1
  Gain1/1 -> beta/1
  Gain/1 -> alpha/1

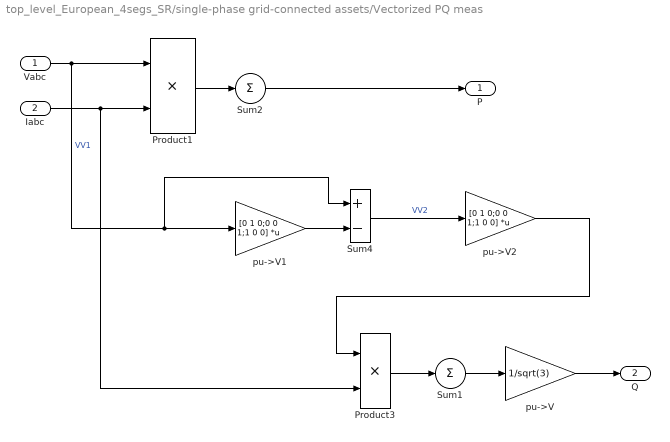
== system top_level_European_4segs_SR/single-phase grid-connected assets/Vectorized PQ meas ==
  Vabc : Inport
  Iabc : Inport  Port=2
  Product1 : Product  InputSameDT=on  SaturateOnIntegerOverflow=on  OutDataTypeStr=Inherit: Same as first input
  Product3 : Product  InputSameDT=on  SaturateOnIntegerOverflow=on  OutDataTypeStr=Inherit: Same as first input
  Sum1 : Sum  Inputs=1  CollapseMode=Specified dimension  InputSameDT=on  SaturateOnIntegerOverflow=on  OutDataTypeStr=Inherit: Same as first input
  Sum2 : Sum  Inputs=1  CollapseMode=Specified dimension  InputSameDT=on  SaturateOnIntegerOverflow=on  OutDataTypeStr=Inherit: Same as first input
  Sum4 : Sum  Inputs=+-  InputSameDT=on  SaturateOnIntegerOverflow=on  OutDataTypeStr=Inherit: Same as first input
  pu->V : Gain  Gain=1/sqrt(3)  SaturateOnIntegerOverflow=on  OutDataTypeStr=Inherit: Same as input  ParamDataTypeStr=Inherit: Same as input
  pu->V1 : Gain  Gain=[0 1 0;0 0 1;1 0 0]  Multiplication=Matrix(K*u)  SaturateOnIntegerOverflow=on  OutDataTypeStr=Inherit: Same as input  ParamDataTypeStr=Inherit: Same as input
  pu->V2 : Gain  Gain=[0 1 0;0 0 1;1 0 0]  Multiplication=Matrix(K*u)  SaturateOnIntegerOverflow=on  OutDataTypeStr=Inherit: Same as input  ParamDataTypeStr=Inherit: Same as input
  P : Outport  VectorParamsAs1DForOutWhenUnconnected=off
  Q : Outport  Port=2  VectorParamsAs1DForOutWhenUnconnected=off
  wires:
  pu->V2/1 -> Product3/1
  Sum4/1 -> pu->V2/1  "VV2"
  pu->V1/1 -> Sum4/2
  Sum2/1 -> P/1
  Iabc/1 -> Product1/2, Product3/2
  Vabc/1 -> Product1/1, pu->V1/1, Sum4/1  "VV1"
  Product1/1 -> Sum2/1
  Product3/1 -> Sum1/1
  Sum1/1 -> pu->V/1
  pu->V/1 -> Q/1

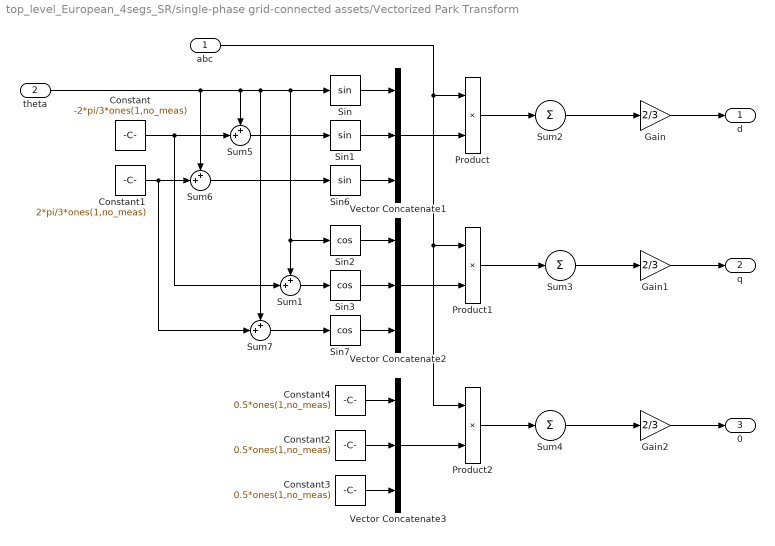
== system top_level_European_4segs_SR/single-phase grid-connected assets/Vectorized Park Transform ==
  abc : Inport
  theta : Inport  Port=2
  Constant : Constant  Value=-2*pi/3*ones(1,no_meas)  VectorParams1D=off  SampleTime=Ts
  Constant1 : Constant  Value=2*pi/3*ones(1,no_meas)  VectorParams1D=off  SampleTime=Ts
  Constant2 : Constant  Value=0.5*ones(1,no_meas)  VectorParams1D=off  SampleTime=Ts
  Constant3 : Constant  Value=0.5*ones(1,no_meas)  VectorParams1D=off  SampleTime=Ts
  Constant4 : Constant  Value=0.5*ones(1,no_meas)  VectorParams1D=off  SampleTime=Ts
  Gain : Gain  Gain=2/3
  Gain1 : Gain  Gain=2/3
  Gain2 : Gain  Gain=2/3
  Product : Product
  Product1 : Product
  Product2 : Product
  Sin : Trigonometry
  Sin1 : Trigonometry
  Sin2 : Trigonometry  Operator=cos
  Sin3 : Trigonometry  Operator=cos
  Sin6 : Trigonometry
  Sin7 : Trigonometry  Operator=cos
  Sum{1,5..7} (4 alike) : Sum  Inputs=++|
  Sum2 : Sum  Inputs=1  CollapseMode=Specified dimension  InputSameDT=on  SaturateOnIntegerOverflow=on  OutDataTypeStr=Inherit: Same as first input
  Sum3 : Sum  Inputs=1  CollapseMode=Specified dimension  InputSameDT=on  SaturateOnIntegerOverflow=on  OutDataTypeStr=Inherit: Same as first input
  Sum4 : Sum  Inputs=1  CollapseMode=Specified dimension  InputSameDT=on  SaturateOnIntegerOverflow=on  OutDataTypeStr=Inherit: Same as first input
  Vector Concatenate1 : Concatenate  NumInputs=3  Mode=Multidimensional array
  Vector Concatenate2 : Concatenate  NumInputs=3  Mode=Multidimensional array
  Vector Concatenate3 : Concatenate  NumInputs=3  Mode=Multidimensional array
  d : Outport  VectorParamsAs1DForOutWhenUnconnected=off
  q : Outport  Port=2  VectorParamsAs1DForOutWhenUnconnected=off
  0 : Outport  Port=3  VectorParamsAs1DForOutWhenUnconnected=off
  wires:
  theta/1 -> Sum7/1, Sin/1, Sum1/1, Sin2/1, Sum5/1, Sum6/1
  Sum7/1 -> Sin7/1
  Sum1/1 -> Sin3/1
  Constant1/1 -> Sum6/2, Sum7/2
  Constant/1 -> Sum5/2, Sum1/2
  Sum6/1 -> Sin6/1
  Sum5/1 -> Sin1/1
  abc/1 -> Product2/1, Product1/1, Product/1
  Sin/1 -> Vector Concatenate1/1
  Sin1/1 -> Vector Concatenate1/2
  Sin3/1 -> Vector Concatenate2/2
  Sin2/1 -> Vector Concatenate2/1
  Constant4/1 -> Vector Concatenate3/1
  Constant2/1 -> Vector Concatenate3/2
  Sin6/1 -> Vector Concatenate1/3
  Sin7/1 -> Vector Concatenate2/3
  Constant3/1 -> Vector Concatenate3/3
  Vector Concatenate3/1 -> Product2/2
  Vector Concatenate2/1 -> Product1/2
  Vector Concatenate1/1 -> Product/2
  Product/1 -> Sum2/1
  Product1/1 -> Sum3/1
  Product2/1 -> Sum4/1
  Sum3/1 -> Gain1/1
  Sum4/1 -> Gain2/1
  Sum2/1 -> Gain/1
  Gain2/1 -> 0/1
  Gain1/1 -> q/1
  Gain/1 -> d/1

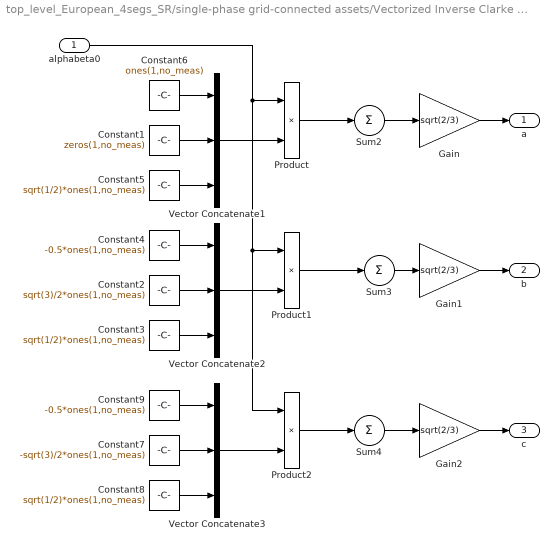
== system top_level_European_4segs_SR/single-phase grid-connected assets/Vectorized Inverse Clarke Transform ==
  alphabeta0 : Inport
  Constant1 : Constant  Value=zeros(1,no_meas)  VectorParams1D=off  SampleTime=Ts
  Constant2 : Constant  Value=sqrt(3)/2*ones(1,no_meas)  VectorParams1D=off  SampleTime=Ts
  Constant3 : Constant  Value=sqrt(1/2)*ones(1,no_meas)  VectorParams1D=off  SampleTime=Ts
  Constant4 : Constant  Value=-0.5*ones(1,no_meas)  VectorParams1D=off  SampleTime=Ts
  Constant5 : Constant  Value=sqrt(1/2)*ones(1,no_meas)  VectorParams1D=off  SampleTime=Ts
  Constant6 : Constant  Value=ones(1,no_meas)  VectorParams1D=off  SampleTime=Ts
  Constant7 : Constant  Value=-sqrt(3)/2*ones(1,no_meas)  VectorParams1D=off  SampleTime=Ts
  Constant8 : Constant  Value=sqrt(1/2)*ones(1,no_meas)  VectorParams1D=off  SampleTime=Ts
  Constant9 : Constant  Value=-0.5*ones(1,no_meas)  VectorParams1D=off  SampleTime=Ts
  Gain : Gain  Gain=sqrt(2/3)
  Gain1 : Gain  Gain=sqrt(2/3)
  Gain2 : Gain  Gain=sqrt(2/3)
  Product : Product
  Product1 : Product
  Product2 : Product
  Sum2 : Sum  Inputs=1  CollapseMode=Specified dimension  InputSameDT=on  SaturateOnIntegerOverflow=on  OutDataTypeStr=Inherit: Same as first input
  Sum3 : Sum  Inputs=1  CollapseMode=Specified dimension  InputSameDT=on  SaturateOnIntegerOverflow=on  OutDataTypeStr=Inherit: Same as first input
  Sum4 : Sum  Inputs=1  CollapseMode=Specified dimension  InputSameDT=on  SaturateOnIntegerOverflow=on  OutDataTypeStr=Inherit: Same as first input
  Vector Concatenate1 : Concatenate  NumInputs=3  Mode=Multidimensional array
  Vector Concatenate2 : Concatenate  NumInputs=3  Mode=Multidimensional array
  Vector Concatenate3 : Concatenate  NumInputs=3  Mode=Multidimensional array
  a : Outport  VectorParamsAs1DForOutWhenUnconnected=off
  b : Outport  Port=2  VectorParamsAs1DForOutWhenUnconnected=off
  c : Outport  Port=3  VectorParamsAs1DForOutWhenUnconnected=off
  wires:
  Constant8/1 -> Vector Concatenate3/3
  Constant7/1 -> Vector Concatenate3/2
  Constant9/1 -> Vector Concatenate3/1
  alphabeta0/1 -> Product/1, Product1/1, Product2/1
  Gain2/1 -> c/1
  Gain1/1 -> b/1
  Gain/1 -> a/1
  Product2/1 -> Sum4/1
  Product1/1 -> Sum3/1
  Product/1 -> Sum2/1
  Vector Concatenate1/1 -> Product/2
  Vector Concatenate2/1 -> Product1/2
  Vector Concatenate3/1 -> Product2/2
  Constant3/1 -> Vector Concatenate2/3
  Constant5/1 -> Vector Concatenate1/3
  Constant4/1 -> Vector Concatenate2/1
  Constant2/1 -> Vector Concatenate2/2
  Constant1/1 -> Vector Concatenate1/2
  Constant6/1 -> Vector Concatenate1/1
  Sum2/1 -> Gain/1
  Sum3/1 -> Gain1/1
  Sum4/1 -> Gain2/1

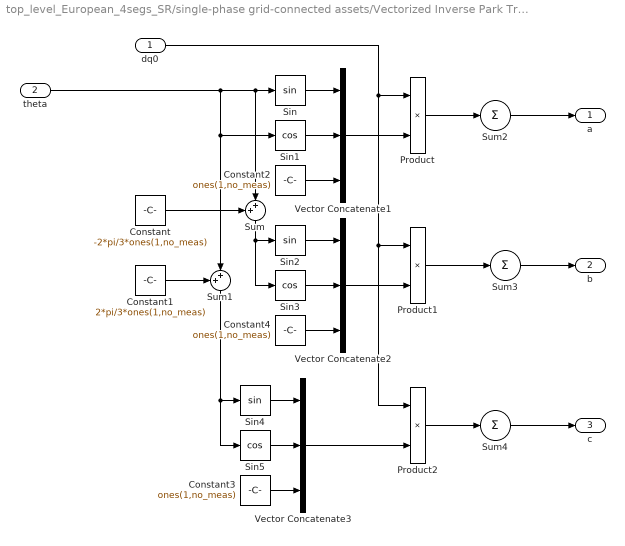
== system top_level_European_4segs_SR/single-phase grid-connected assets/Vectorized Inverse Park Transform ==
  dq0 : Inport
  theta : Inport  Port=2
  Constant : Constant  Value=-2*pi/3*ones(1,no_meas)  VectorParams1D=off  SampleTime=Ts
  Constant1 : Constant  Value=2*pi/3*ones(1,no_meas)  VectorParams1D=off  SampleTime=Ts
  Constant2 : Constant  Value=ones(1,no_meas)  VectorParams1D=off  SampleTime=Ts
  Constant3 : Constant  Value=ones(1,no_meas)  VectorParams1D=off  SampleTime=Ts
  Constant4 : Constant  Value=ones(1,no_meas)  VectorParams1D=off  SampleTime=Ts
  Product : Product
  Product1 : Product
  Product2 : Product
  Sin : Trigonometry
  Sin1 : Trigonometry  Operator=cos
  Sin2 : Trigonometry
  Sin3 : Trigonometry  Operator=cos
  Sin4 : Trigonometry
  Sin5 : Trigonometry  Operator=cos
  Sum : Sum  Inputs=++|
  Sum1 : Sum  Inputs=++|
  Sum2 : Sum  Inputs=1  CollapseMode=Specified dimension  InputSameDT=on  SaturateOnIntegerOverflow=on  OutDataTypeStr=Inherit: Same as first input
  Sum3 : Sum  Inputs=1  CollapseMode=Specified dimension  InputSameDT=on  SaturateOnIntegerOverflow=on  OutDataTypeStr=Inherit: Same as first input
  Sum4 : Sum  Inputs=1  CollapseMode=Specified dimension  InputSameDT=on  SaturateOnIntegerOverflow=on  OutDataTypeStr=Inherit: Same as first input
  Vector Concatenate1 : Concatenate  NumInputs=3  Mode=Multidimensional array
  Vector Concatenate2 : Concatenate  NumInputs=3  Mode=Multidimensional array
  Vector Concatenate3 : Concatenate  NumInputs=3  Mode=Multidimensional array
  a : Outport  VectorParamsAs1DForOutWhenUnconnected=off
  b : Outport  Port=2  VectorParamsAs1DForOutWhenUnconnected=off
  c : Outport  Port=3  VectorParamsAs1DForOutWhenUnconnected=off
  wires:
  Product2/1 -> Sum4/1
  Product1/1 -> Sum3/1
  Product/1 -> Sum2/1
  Vector Concatenate1/1 -> Product/2
  Vector Concatenate2/1 -> Product1/2
  Vector Concatenate3/1 -> Product2/2
  Constant3/1 -> Vector Concatenate3/3
  Constant4/1 -> Vector Concatenate2/3
  Constant2/1 -> Vector Concatenate1/3
  Sin5/1 -> Vector Concatenate3/2
  Sin4/1 -> Vector Concatenate3/1
  Sum1/1 -> Sin5/1, Sin4/1
  Constant1/1 -> Sum1/1
  Constant/1 -> Sum/1
  Sum/1 -> Sin2/1, Sin3/1
  Sin2/1 -> Vector Concatenate2/1
  Sin3/1 -> Vector Concatenate2/2
  Sin1/1 -> Vector Concatenate1/2
  Sin/1 -> Vector Concatenate1/1
  dq0/1 -> Product/1, Product1/1, Product2/1
  theta/1 -> Sum/2, Sin/1, Sum1/2, Sin1/1
  Sum2/1 -> a/1
  Sum3/1 -> b/1
  Sum4/1 -> c/1
